simulink model "Capacitive_Balancing"  (R2024b)
settings: Solver=VariableStepAuto  StartTime=0.0  StopTime=10000  RelTol=1e-3
undefined symbols (not defined in the file): Ion, Lithium
libraries: spsIdealSwitchLib x4, spsBatteryLib x2, spsPWMGenerator2LevelLib x1, spsSeriesRLCBranchLib x1, sps_lib x1
settings Model: Creator=yeswa  LastModifiedBy=yeswa

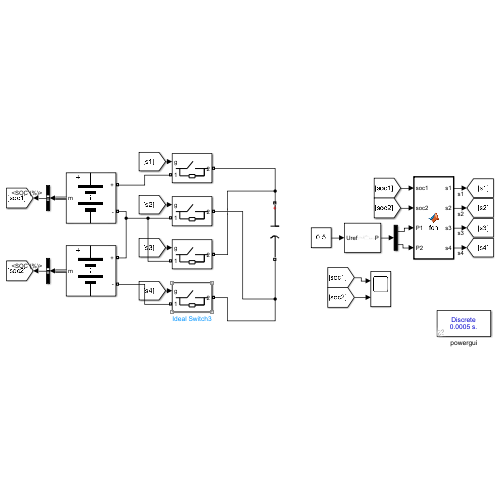
[thumbnail: Simulink's stored preview of the top-level diagram]
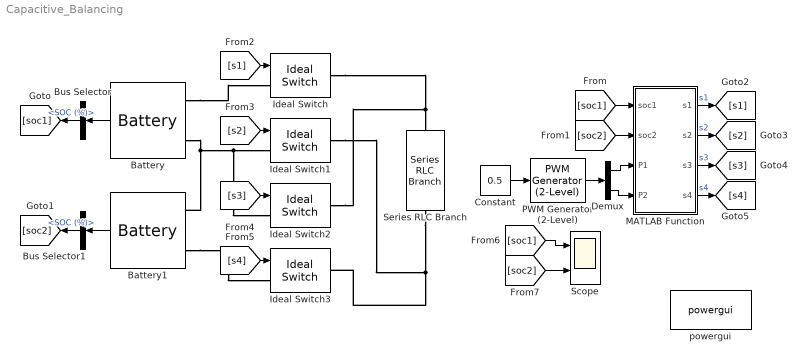
== system Capacitive_Balancing ==
  Battery : spsBatteryLib/Battery  BatType=Lithium-Ion  NomV=3.7  NomQ=5.4  SOC=50  Batt_Tr=30  PresetModel=on  MaxQ=5.4  MinV=2.775  FullV=4.3068  Dis_rate=2.3478  R=0.0068519  Normal_OP=4.8835  expZone="[3.9974      0.2653]"
  Battery1 : spsBatteryLib/Battery  BatType=Lithium-Ion  NomV=3.7  NomQ=5.4  SOC=40  Batt_Tr=30  PresetModel=on  MaxQ=5.4  MinV=2.775  FullV=4.3068  Dis_rate=2.3478  R=0.0068519  Normal_OP=4.8835  expZone="[3.9974      0.2653]"
  Bus Selector : BusSelector  OutputSignals=SOC (%)
  Bus Selector1 : BusSelector  OutputSignals=SOC (%)
  Constant : Constant  Value=0.5
  Demux : Demux  Outputs=2
  Ideal Switch{,1..3} (4 alike) : spsIdealSwitchLib/Ideal Switch  Ron=0.001  Lon=0  IC=0  Rs=1e5  Cs=inf  Measurements=off
  MATLAB Function : MATLAB Function  TreatAsAtomicUnit=on
  PWM Generator (2-Level) : spsPWMGenerator2LevelLib/PWM Generator (2-Level)  ModulatorType=Single-phase half-bridge (2 pulses)  ModulatorMode=Unsynchronized  Fc=200  Pc=0  nF=27  MinMax="[ -1  1 ]"  SamplingTechnique=Natural  ModulatingSignals=off  m=0.8  Freq=60  Phase=0  Ts=0  ShowCarrierOutport=off
  Scope : Scope  NumInputPorts=2
  Series RLC Branch : spsSeriesRLCBranchLib/Series RLC Branch  LConnTagsString=__new0  RConnTagsString=__new0  BranchType=C  Resistance=1  Inductance=1e-3  SetiL0=off  InitialCurrent=0  Capacitance=10  Setx0=off  InitialVoltage=0  Measurements=None
  powergui : sps_lib/powergui  Priority=1  SimulationMode=Discrete  SampleTime=5e-4  frequency=60  Iterations=50  frequencyindice=0  Pbase=100e6  ErrMax=1e-4  UnitsV=kV  UnitsW=MW  buscounter=0  FunctionMessages=off  echomessages=off  EnableUseOfTLC=off  CurrentSourceSwitches=off  DisableSnubberDevices=off  DisableRonSwitches=off  DisableVfSwitches=off  DisplayEquations=off  AutomaticDiscreteSolvers=off  SolverType=Tustin/Backward Euler (TBE)  Interpol=off  ExternalGateDelay=off  methode=off  Ts=100  x0status=blocks  SPID=on  SwTol=0  HookPort=off  NonlinearTolerance=1e-4  nMaxIteration=100  ContinueOnMaxIteration=off  RestoreLinks=warning  ResistiveCurrentMeasurement=off  Frange=[0:2:500]  Ylog=off  Xlog=on  ShowGrid=off  save=off  variable=ZData  structure=0  ZoomFFT=off  StartTime=0.0  cycles=1  DisplayStyle=1  fundamental=60  FreqAxis=off  MaxFrequency=1000  frequencyindicesteady=1  RmsSteady=1  display=off
  wires:
  Battery/1 -> Bus Selector/1
  Bus Selector/1 -> [soc1]  "<SOC (%)>"
  Bus Selector1/1 -> [soc2]  "<SOC (%)>"
  Battery1/1 -> Bus Selector1/1
  [soc1] -> MATLAB Function/1(soc1)
  [soc2] -> MATLAB Function/2(soc2)
  Constant/1 -> PWM Generator (2-Level)/1
  PWM Generator (2-Level)/1 -> Demux/1
  [s1] -> Ideal Switch/1
  [s2] -> Ideal Switch1/1
  [s3] -> Ideal Switch2/1
  [s4] -> Ideal Switch3/1
  [soc2] -> Scope/2
  [soc1] -> Scope/1
  MATLAB Function/1(s1) -> [s1]  "s1"
  MATLAB Function/2(s2) -> [s2]  "s2"
  MATLAB Function/3(s3) -> [s3]  "s3"
  MATLAB Function/4(s4) -> [s4]  "s4"
  Demux/1 -> MATLAB Function/3(P1)
  Demux/2 -> MATLAB Function/4(P2)
  connections:
  Battery/LConn2 -- Ideal Switch2/LConn1 -- Ideal Switch1/LConn1 -- Battery1/LConn1
  Battery/LConn1 -- Ideal Switch/LConn1
  Battery1/LConn2 -- Ideal Switch3/LConn1
  Ideal Switch/RConn1 -- Series RLC Branch/LConn1 -- Ideal Switch2/RConn1
  Ideal Switch1/RConn1 -- Series RLC Branch/RConn1 -- Ideal Switch3/RConn1

== matlab function Capacitive_Balancing/MATLAB Function ==
  data: soc1 input; s1 output; soc2 input; P1 input; P2 input; s2 output; s3 output; s4 output
function [s1,s2,s3,s4] = fcn(soc1,soc2,P1,P2)

% Threshold for SOC difference (tune as needed, e.g. 0.01 = 1%)
threshold = 0.01;  

if abs(soc1 - soc2) > threshold
    % Enable balancing (capacitor charge/discharge cycle)
    s1 = P1;
    s2 = P1;
    s3 = P2;
    s4 = P2;
else
    % SOCs close enough → no balancing
    s1 = 0;
    s2 = 0;
    s3 = 0;
    s4 = 0;
end

end
